simulink model "kalman_filter_try"  (R2024a)
settings: Solver=VariableStepAuto  StartTime=0.0  StopTime=10.0  RelTol=1e-3

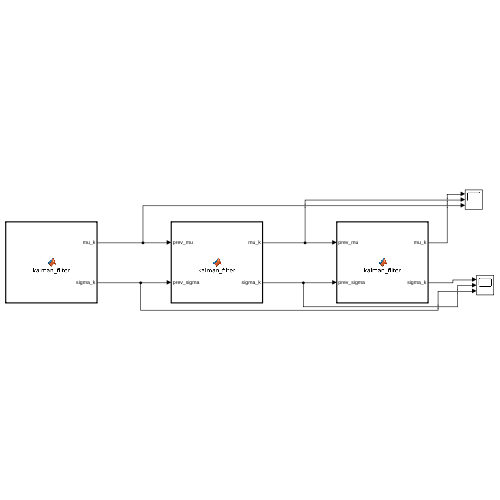
[thumbnail: Simulink's stored preview of the top-level diagram]
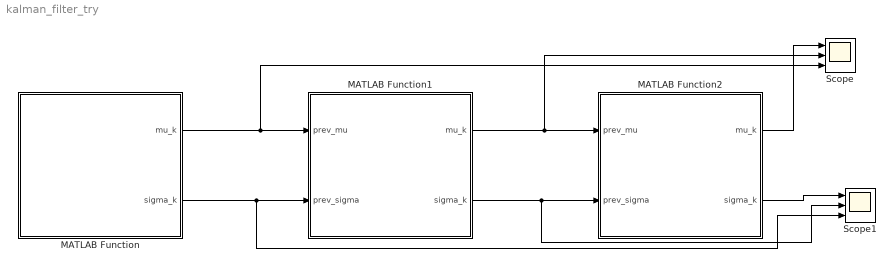
== system kalman_filter_try ==
  MATLAB Function : MATLAB Function  TreatAsAtomicUnit=on
  MATLAB Function1 : MATLAB Function  TreatAsAtomicUnit=on
  MATLAB Function2 : MATLAB Function  TreatAsAtomicUnit=on
  Scope : Scope  NumInputPorts=3
  Scope1 : Scope  NumInputPorts=3
  wires:
  MATLAB Function/1(mu_k) -> Scope/3, MATLAB Function1/1(prev_mu)
  MATLAB Function/2(sigma_k) -> Scope1/3, MATLAB Function1/2(prev_sigma)
  MATLAB Function1/1(mu_k) -> Scope/2, MATLAB Function2/1(prev_mu)
  MATLAB Function1/2(sigma_k) -> Scope1/2, MATLAB Function2/2(prev_sigma)
  MATLAB Function2/1(mu_k) -> Scope/1
  MATLAB Function2/2(sigma_k) -> Scope1/1

== matlab function kalman_filter_try/MATLAB Function1 ==
  data: mu_k output; sigma_k output; prev_mu input; prev_sigma input
function [mu_k,sigma_k]= kalman_filter(prev_mu, prev_sigma)
mu=prev_mu;
init_covar=prev_sigma;
landmark=[3;4];
Vk=1;
Wk=1;
delta_t=.1;
Qk=[.5 .01 .01; .01 .5 .01; .01 .01 .2];
Rk=[.1 0; 0 .02];
Z=[4.72 .72]';
I=[1 0 0; 0 1 0; 0 0 1];

%posicion estimada
step=[delta_t*Vk*cos(mu(3)); delta_t*Vk*sin(mu(3)); delta_t*Wk];
mu_hat=mu+step;

%linelaizacion
Hk=[1 0 -delta_t*Vk*sin(mu(3)); 1 0 delta_t*Vk*cos(mu(3)); 0 0 1];

%propagacion de incertidumbre
sigma_hat=Hk*init_covar*Hk'+Qk;

%modelo de observacion
delta_x=landmark(1)-mu_hat(1);
delta_y=landmark(2)-mu_hat(2);
p=(delta_x*delta_x)+(delta_y*delta_y);

Z_hat=[sqrt(p); atan2(delta_y,delta_x)-mu_hat(3)];

%linealizacion modelo de observacion
Gk=[-delta_x/sqrt(p) -delta_y/sqrt(p) 0; delta_y/p -delta_x/p -1];

%incertidumbre de la medicion 
Zk=Gk*sigma_hat*Gk'+Rk;

%ganancia de kalman
K=sigma_hat*Gk'*inv(Zk);

%posicion real usando observacion
mu_k=mu_hat+K*(Z-Z_hat);

%covarianza
sigma_k=(I-K*Gk)*Qk;

== matlab function kalman_filter_try/MATLAB Function ==
  data: mu_k output; sigma_k output
function [mu_k,sigma_k]= kalman_filter
mu=[0;0;0];
init_covar=[0 0 0; 0 0 0; 0 0 0];
landmark=[3;4];
Vk=1;
Wk=1;
delta_t=.1;
Qk=[.5 .01 .01; .01 .5 .01; .01 .01 .2];
Rk=[.1 0; 0 .02];
Z=[4.87 .8]';
I=[1 0 0; 0 1 0; 0 0 1];

%posicion estimada
step=[delta_t*Vk*cos(mu(3)); delta_t*Vk*sin(mu(3)); delta_t*Wk];
mu_hat=mu+step;

%linelaizacion
Hk=[1 0 -delta_t*Vk*sin(mu(3)); 1 0 delta_t*Vk*cos(mu(3)); 0 0 1];

%propagacion de incertidumbre
sigma_hat=Hk*init_covar*Hk'+Qk;

%modelo de observacion
delta_x=landmark(1)-mu_hat(1);
delta_y=landmark(2)-mu_hat(2);
p=(delta_x*delta_x)+(delta_y*delta_y);

Z_hat=[sqrt(p); atan2(delta_y,delta_x)-mu_hat(3)];

%linealizacion modelo de observacion
Gk=[-delta_x/sqrt(p) -delta_y/sqrt(p) 0; delta_y/p -delta_x/p -1];

%incertidumbre de la medicion 
Zk=Gk*sigma_hat*Gk'+Rk;

%ganancia de kalman
K=sigma_hat*Gk'*inv(Zk);

%posicion real usando observacion
mu_k=mu_hat+K*(Z-Z_hat);

%covarianza
sigma_k=(I-K*Gk)*Qk;

== matlab function kalman_filter_try/MATLAB Function2 ==
  data: mu_k output; sigma_k output; prev_mu input; prev_sigma input
function [mu_k,sigma_k]= kalman_filter(prev_mu,prev_sigma)
mu=prev_mu;
init_covar=prev_sigma;
landmark=[3;4];
Vk=1;
Wk=1;
delta_t=.1;
Qk=[.5 .01 .01; .01 .5 .01; .01 .01 .2];
Rk=[.1 0; 0 .02];
Z=[4.69 .65]';
I=[1 0 0; 0 1 0; 0 0 1];

%posicion estimada
step=[delta_t*Vk*cos(mu(3)); delta_t*Vk*sin(mu(3)); delta_t*Wk];
mu_hat=mu+step;

%linelaizacion
Hk=[1 0 -delta_t*Vk*sin(mu(3)); 1 0 delta_t*Vk*cos(mu(3)); 0 0 1];

%propagacion de incertidumbre
sigma_hat=Hk*init_covar*Hk'+Qk;

%modelo de observacion
delta_x=landmark(1)-mu_hat(1);
delta_y=landmark(2)-mu_hat(2);
p=(delta_x*delta_x)+(delta_y*delta_y);

Z_hat=[sqrt(p); atan2(delta_y,delta_x)-mu_hat(3)];

%linealizacion modelo de observacion
Gk=[-delta_x/sqrt(p) -delta_y/sqrt(p) 0; delta_y/p -delta_x/p -1];

%incertidumbre de la medicion 
Zk=Gk*sigma_hat*Gk'+Rk;

%ganancia de kalman
K=sigma_hat*Gk'*inv(Zk);

%posicion real usando observacion
mu_k=mu_hat+K*(Z-Z_hat);

%covarianza
sigma_k=(I-K*Gk)*Qk;
